simulink model "BBB_GPIO_Read_Test_rev1"  (R2013a)
settings: Solver=FixedStepDiscrete  StartTime=0.0  StopTime=inf  FixedStep=0.01  RelTol=1e-3
libraries: simulink x5
settings Model: SimulationMode=external  ExtModeTrigDuration=100  Creator=rdustinkahawita  LastModifiedBy=rdustinkahawita
settings OptimizationCC: OptimizeModelRefInitCode=on  LifeSpan=1
settings DebuggingCC: SolverPrmCheckMsg=none  StrictBusMsg=Warning
settings HardwareCC: ProdLargestAtomicInteger=Long  ProdLargestAtomicFloat=Double  ProdEndianess=LittleEndian  ProdHWDeviceType=ARM Compatible->ARM Cortex
settings RTWCC: SystemTargetFile=realtime.tlc  GenerateMakefile=off  TemplateMakefile=realtime.tmf  Description=Run on Target Hardware  RTWVerbose=off  ProcessScript=realtime_make_rtw_hook
settings STFCustomTargetCC: TargetLibSuffix=.a  GenerateSampleERTMain=on  ERTCustomFileBanners=on  SupportNonInlinedSFcns=off  SupportVariableSizeSignals=on  MATLABClassNameForMDSCustomization=Simulink.SoftwareTarget.ERTCustomization  SystemTargetFile=realtime.tlc
settings ERTTargetCC: ParMdlRefBuildCompliant=off  CompOptLevelCompliant=off  ConcurrentExecutionCompliant=off  CombineOutputUpdateFcns=off  ERTFirstTimeCompliant=off  SupportContinuousTime=on  SupportVariableSizeSignals=on  ModelStepFunctionPrototypeControlCompliant=off  CPPClassGenCompliant=off  ExtMode=on  ExtModeMexArgs='192.168.7.2' 0 17725  ERTSrcFileBannerTemplate=realtime_code_template.cgt  ERTHdrFileBannerTemplate=realtime_code_template.cgt  ERTDataSrcFileTemplate=realtime_code_template.cgt  ERTDataHdrFileTemplate=realtime_code_template.cgt  ERTCustomFileTemplate=realtime_file_process.tlc

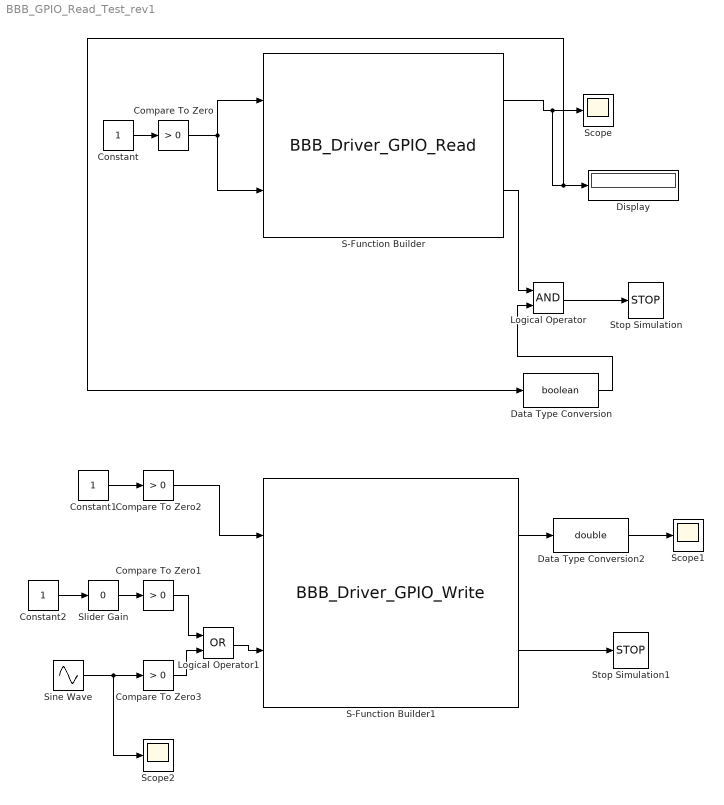
== system BBB_GPIO_Read_Test_rev1 ==
  Compare To Zero{,1..3} (4 alike) : simulink/Logic and Bit Operations/Compare To Zero  relop=>  OutDataTypeStr=boolean
  Constant : Constant
  Constant1 : Constant
  Constant2 : Constant
  Data Type Conversion : DataTypeConversion  OutMin=[0]  OutMax=[1]  OutDataTypeStr=boolean  RndMeth=Round
  Data Type Conversion2 : DataTypeConversion  OutMin=[0]  OutMax=[1]  OutDataTypeStr=double  RndMeth=Round
  Display : Display
  Logical Operator : Logic  AllPortsSameDT=off  OutDataTypeStr=boolean
  Logical Operator1 : Logic  Operator=OR  AllPortsSameDT=off  OutDataTypeStr=boolean
  S-Function Builder : S-Function  InitFcn=try, set_param(gcb,'FunctionName','BBB_Driver_GPIO_Read'), end  FunctionName=BBB_Driver_GPIO_Read  Parameters=uint16(1),uint16(4)  SFunctionModules=BBB_Driver_GPIO_Read_wrapper  EnableBusSupport=off  mask(S-Function Builder){}
      mask help: Simulink:masks:SFunctionBuilder_MD
      mask init:
      | val = [[.9  0.75 0.75 1 1 .9 .9 1]',[1 1 0.75 0.75 .9 .9 1 .9]'];try , sys = get_param(gcb,'SfunBuilderFcnName');if isempty(sys), sys = get_param(gcb,'FunctionName'); end,catch, sys = get_param(gcb,'FunctionName'); end
      settings: CopyFcn=set_param(gcbh,'LinkStatus','none')  PreSaveFcn=try, set_param(gcb,'FunctionName','BBB_Driver_GPIO_Read'), end  OpenFcn=sfunctionwizard(gcbh)
      mask Display: plot(val(:,1),val(:,2)),disp(sys), port_label('input',1,'inGPIO_Read_Enable'), port_label('input',2,'inGPIO_Read'), port_label('output',1,'outGPIO_ReadValue'), port_label('output',2,'outSimStop')
  S-Function Builder1 : S-Function  InitFcn=try, set_param(gcb,'FunctionName','BBB_Driver_GPIO_Write'), end  FunctionName=BBB_Driver_GPIO_Write  Parameters=uint16(3),uint16(4)  SFunctionModules=BBB_Driver_GPIO_Write_wrapper  EnableBusSupport=off  mask(S-Function Builder){}
      mask help: Simulink:masks:SFunctionBuilder_MD
      mask init: same as BBB_GPIO_Read_Test_rev1/S-Function Builder
      settings: CopyFcn=set_param(gcbh,'LinkStatus','none')  PreSaveFcn=try, set_param(gcb,'FunctionName','BBB_Driver_GPIO_Write'), end  OpenFcn=sfunctionwizard(gcbh)
      mask Display: plot(val(:,1),val(:,2)),disp(sys), port_label('input',1,'inGPIO_Write_Enable'), port_label('input',2,'inGPIO_Write'), port_label('output',1,'outGPIO_WriteValue'), port_label('output',2,'outSimStop')
  Scope : Scope
  Scope1 : Scope
  Scope2 : Scope
      settings: SaveName=ScopeData2
  Sine Wave : Sin  Frequency=4
  Slider Gain : simulink/Math Operations/Slider Gain  low=0  gain=0  high=1
  Stop Simulation : Stop
  Stop Simulation1 : Stop
  wires:
  Compare To Zero/1 -> S-Function Builder/1, S-Function Builder/2
  S-Function Builder/1 -> Data Type Conversion/1, Display/1, Scope/1
  Constant/1 -> Compare To Zero/1
  Data Type Conversion/1 -> Logical Operator/2
  S-Function Builder/2 -> Logical Operator/1
  Logical Operator/1 -> Stop Simulation/1
  Constant1/1 -> Compare To Zero2/1
  Compare To Zero2/1 -> S-Function Builder1/1
  S-Function Builder1/1 -> Data Type Conversion2/1
  Data Type Conversion2/1 -> Scope1/1
  S-Function Builder1/2 -> Stop Simulation1/1
  Slider Gain/1 -> Compare To Zero1/1
  Constant2/1 -> Slider Gain/1
  Logical Operator1/1 -> S-Function Builder1/2
  Compare To Zero1/1 -> Logical Operator1/1
  Compare To Zero3/1 -> Logical Operator1/2
  Sine Wave/1 -> Scope2/1, Compare To Zero3/1
